simulink library "GenericINSLibrary"  (R2020b)
settings: Solver=VariableStepAuto  StartTime=0.0  StopTime=10.0  RelTol=1e-3
libraries: simulink x44
(part 3 of 6)

== system GenericINSLibrary/Empty Bus Sensor Fusion No Bias Estimation/GNSS6 ==
  Bus Creator : BusCreator  Inputs=1
  Bus Creator1 : BusCreator  Inputs=3
  Bus Creator2 : BusCreator  Inputs=3
  Bus Creator3 : BusCreator  Inputs=4
  Constant71 : Constant  Value=[0;0;0]  OutDataTypeStr=double
  Constant72 : Constant  OutDataTypeStr=double
  Constant73 : Constant  OutDataTypeStr=double
  Constant74 : Constant  OutDataTypeStr=double
  Constant{75..78} (4 alike) : Constant  Value=0  OutDataTypeStr=double
  Signal Specification : SignalSpecification  OutDataTypeStr=double  Unit=m  Dimensions=3
  Signal Specification{1..3,7} (4 alike) : SignalSpecification  OutDataTypeStr=double  Unit=m  Dimensions=1
  Signal Specification4 : SignalSpecification  OutDataTypeStr=double  Unit=s  Dimensions=1
  Signal Specification5 : SignalSpecification  OutDataTypeStr=double  Unit=rad  Dimensions=1
  Signal Specification6 : SignalSpecification  OutDataTypeStr=double  Unit=rad  Dimensions=1
  busGNSS : Outport
  wires:
  Bus Creator1/1 -> busGNSS/1
  Signal Specification4/1 -> Bus Creator3/1  "timestamp"
  Constant75/1 -> Signal Specification4/1
  Signal Specification/1 -> Bus Creator/1  "positionBodyToSensor"
  Signal Specification2/1 -> Bus Creator2/2  "east"
  Constant74/1 -> Signal Specification3/1
  Bus Creator/1 -> Bus Creator1/1  "alignment"
  Signal Specification3/1 -> Bus Creator2/3  "down"
  Bus Creator3/1 -> Bus Creator1/3  "measurement"
  Bus Creator2/1 -> Bus Creator1/2  "standardDeviation"
  Signal Specification5/1 -> Bus Creator3/2  "latitude"
  Constant78/1 -> Signal Specification7/1
  Signal Specification7/1 -> Bus Creator3/4  "altitude"
  Constant73/1 -> Signal Specification2/1
  Constant71/1 -> Signal Specification/1
  Constant76/1 -> Signal Specification5/1
  Constant77/1 -> Signal Specification6/1
  Signal Specification1/1 -> Bus Creator2/1  "north"
  Constant72/1 -> Signal Specification1/1
  Signal Specification6/1 -> Bus Creator3/3  "longitude"

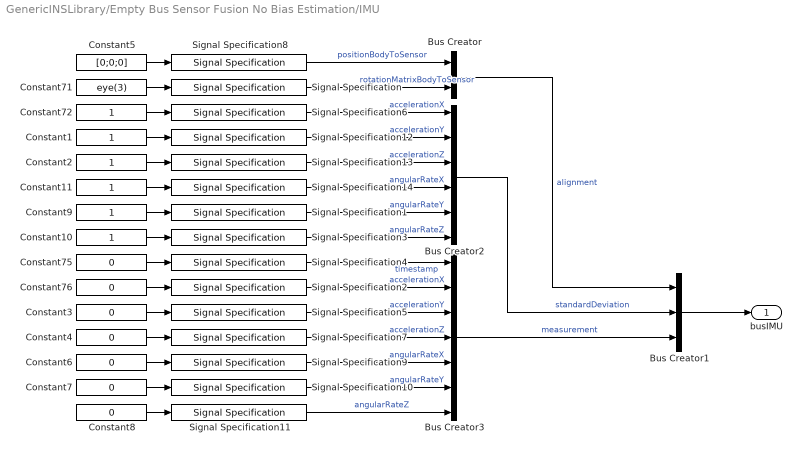
== system GenericINSLibrary/Empty Bus Sensor Fusion No Bias Estimation/IMU ==
  Bus Creator : BusCreator  Inputs=2
  Bus Creator1 : BusCreator  Inputs=3
  Bus Creator2 : BusCreator  Inputs=6
  Bus Creator3 : BusCreator  Inputs=7
  Constant{1..2,9..11,72} (6 alike) : Constant  OutDataTypeStr=double
  Constant{3..4,6..8,75..76} (7 alike) : Constant  Value=0  OutDataTypeStr=double
  Constant5 : Constant  Value=[0;0;0]  OutDataTypeStr=double
  Constant71 : Constant  Value=eye(3)  OutDataTypeStr=double
  Signal Specification : SignalSpecification  OutDataTypeStr=double  Dimensions=[3 3]
  Signal Specification{1,3,9..11,14} (6 alike) : SignalSpecification  OutDataTypeStr=double  Unit=rad/s  Dimensions=1
  Signal Specification{2,5..7,12..13} (6 alike) : SignalSpecification  OutDataTypeStr=double  Unit=m/s^2  Dimensions=1
  Signal Specification4 : SignalSpecification  OutDataTypeStr=double  Unit=s  Dimensions=1
  Signal Specification8 : SignalSpecification  OutDataTypeStr=double  Unit=m  Dimensions=3
  busIMU : Outport
  wires:
  Constant4/1 -> Signal Specification7/1
  Constant2/1 -> Signal Specification13/1
  Bus Creator1/1 -> busIMU/1
  Signal Specification4/1 -> Bus Creator3/1  "timestamp"
  Constant75/1 -> Signal Specification4/1
  Signal Specification/1 -> Bus Creator/2  "rotationMatrixBodyToSensor"
  Bus Creator/1 -> Bus Creator1/1  "alignment"
  Bus Creator3/1 -> Bus Creator1/3  "measurement"
  Bus Creator2/1 -> Bus Creator1/2  "standardDeviation"
  Constant71/1 -> Signal Specification/1
  Constant76/1 -> Signal Specification2/1
  Constant72/1 -> Signal Specification6/1
  Signal Specification2/1 -> Bus Creator3/2  "accelerationX"
  Constant1/1 -> Signal Specification12/1
  Constant3/1 -> Signal Specification5/1
  Signal Specification8/1 -> Bus Creator/1  "positionBodyToSensor"
  Constant5/1 -> Signal Specification8/1
  Signal Specification5/1 -> Bus Creator3/3  "accelerationY"
  Signal Specification7/1 -> Bus Creator3/4  "accelerationZ"
  Constant6/1 -> Signal Specification9/1
  Signal Specification9/1 -> Bus Creator3/5  "angularRateX"
  Constant7/1 -> Signal Specification10/1
  Constant8/1 -> Signal Specification11/1
  Signal Specification10/1 -> Bus Creator3/6  "angularRateY"
  Signal Specification11/1 -> Bus Creator3/7  "angularRateZ"
  Signal Specification3/1 -> Bus Creator2/6  "angularRateZ"
  Signal Specification1/1 -> Bus Creator2/5  "angularRateY"
  Signal Specification14/1 -> Bus Creator2/4  "angularRateX"
  Signal Specification13/1 -> Bus Creator2/3  "accelerationZ"
  Signal Specification12/1 -> Bus Creator2/2  "accelerationY"
  Signal Specification6/1 -> Bus Creator2/1  "accelerationX"
  Constant9/1 -> Signal Specification1/1
  Constant11/1 -> Signal Specification14/1
  Constant10/1 -> Signal Specification3/1

== system GenericINSLibrary/Empty Bus Sensor Fusion No Bias Estimation/InitialStandardDeviation ==
  Bus Creator2 : BusCreator  Inputs=9
  Constant{86..94} (9 alike) : Constant  OutDataTypeStr=double
  Signal Specification16 : SignalSpecification  OutDataTypeStr=double  Unit=m/s  Dimensions=1
  Signal Specification23 : SignalSpecification  OutDataTypeStr=double  Unit=m/s  Dimensions=1
  Signal Specification24 : SignalSpecification  OutDataTypeStr=double  Unit=m/s  Dimensions=1
  Signal Specification{25..27,29..30} (5 alike) : SignalSpecification  OutDataTypeStr=double  Unit=rad  Dimensions=1
  Signal Specification28 : SignalSpecification  OutDataTypeStr=double  Unit=m  Dimensions=1
  initialStandardDeviation : Outport
  wires:
  Signal Specification25/1 -> Bus Creator2/7  "orientationVectorX"
  Signal Specification23/1 -> Bus Creator2/5  "velocityV"
  Constant90/1 -> Signal Specification29/1
  Constant94/1 -> Signal Specification30/1
  Constant89/1 -> Signal Specification25/1
  Signal Specification16/1 -> Bus Creator2/4  "velocityU"
  Signal Specification26/1 -> Bus Creator2/1  "latitude"
  Constant88/1 -> Signal Specification24/1
  Signal Specification27/1 -> Bus Creator2/2  "longitude"
  Constant87/1 -> Signal Specification23/1
  Signal Specification24/1 -> Bus Creator2/6  "velocityW"
  Constant86/1 -> Signal Specification16/1
  Constant93/1 -> Signal Specification28/1
  Constant92/1 -> Signal Specification27/1
  Constant91/1 -> Signal Specification26/1
  Signal Specification28/1 -> Bus Creator2/3  "altitude"
  Bus Creator2/1 -> initialStandardDeviation/1  "standardDeviation"
  Signal Specification30/1 -> Bus Creator2/9  "orientationVectorZ"
  Signal Specification29/1 -> Bus Creator2/8  "orientationVectorY"

== system GenericINSLibrary/Empty Bus Sensor Fusion No Bias Estimation/InitialState ==
  Bus Creator1 : BusCreator  Inputs=9
  Constant{71..79} (9 alike) : Constant  Value=0  OutDataTypeStr=double
  Signal Specification1 : SignalSpecification  OutDataTypeStr=double  Unit=m/s  Dimensions=1
  Signal Specification2 : SignalSpecification  OutDataTypeStr=double  Unit=m/s  Dimensions=1
  Signal Specification3 : SignalSpecification  OutDataTypeStr=double  Unit=m/s  Dimensions=1
  Signal Specification{4..6,8..9} (5 alike) : SignalSpecification  OutDataTypeStr=double  Unit=rad  Dimensions=1
  Signal Specification7 : SignalSpecification  OutDataTypeStr=double  Unit=m  Dimensions=1
  initialState : Outport
  wires:
  Signal Specification4/1 -> Bus Creator1/7  "roll"
  Signal Specification6/1 -> Bus Creator1/2  "longitude"
  Constant73/1 -> Signal Specification3/1
  Constant79/1 -> Signal Specification9/1
  Signal Specification9/1 -> Bus Creator1/9  "yaw"
  Signal Specification2/1 -> Bus Creator1/5  "velocityV"
  Constant71/1 -> Signal Specification1/1
  Constant75/1 -> Signal Specification8/1
  Signal Specification5/1 -> Bus Creator1/1  "latitude"
  Signal Specification7/1 -> Bus Creator1/3  "altitude"
  Signal Specification8/1 -> Bus Creator1/8  "pitch"
  Signal Specification3/1 -> Bus Creator1/6  "velocityW"
  Signal Specification1/1 -> Bus Creator1/4  "velocityU"
  Constant72/1 -> Signal Specification2/1
  Constant77/1 -> Signal Specification6/1
  Constant76/1 -> Signal Specification5/1
  Bus Creator1/1 -> initialState/1
  Constant78/1 -> Signal Specification7/1
  Constant74/1 -> Signal Specification4/1

== system GenericINSLibrary/Empty Bus Sensor Fusion No Bias Estimation/SOG1 ==
  Bus Creator : BusCreator  Inputs=1
  Bus Creator1 : BusCreator  Inputs=3
  Bus Creator2 : BusCreator  Inputs=1
  Bus Creator3 : BusCreator  Inputs=2
  Constant71 : Constant  Value=[0;0;0]  OutDataTypeStr=double
  Constant72 : Constant  OutDataTypeStr=double
  Constant75 : Constant  Value=0  OutDataTypeStr=double
  Constant76 : Constant  Value=0  OutDataTypeStr=double
  Signal Specification : SignalSpecification  OutDataTypeStr=double  Unit=m  Dimensions=3
  Signal Specification1 : SignalSpecification  OutDataTypeStr=double  Unit=m/s  Dimensions=1
  Signal Specification2 : SignalSpecification  OutDataTypeStr=double  Unit=m/s  Dimensions=1
  Signal Specification4 : SignalSpecification  OutDataTypeStr=double  Unit=s  Dimensions=1
  busSOG : Outport
  wires:
  Bus Creator1/1 -> busSOG/1
  Signal Specification4/1 -> Bus Creator3/1  "timestamp"
  Constant75/1 -> Signal Specification4/1
  Signal Specification/1 -> Bus Creator/1  "positionBodyToSensor"
  Bus Creator/1 -> Bus Creator1/1  "alignment"
  Bus Creator3/1 -> Bus Creator1/3  "measurement"
  Bus Creator2/1 -> Bus Creator1/2  "standardDeviation"
  Constant71/1 -> Signal Specification/1
  Constant76/1 -> Signal Specification2/1
  Signal Specification1/1 -> Bus Creator2/1  "speedOverGround"
  Constant72/1 -> Signal Specification1/1
  Signal Specification2/1 -> Bus Creator3/2  "speedOverGround"

== system GenericINSLibrary/Empty Bus Sensor Fusion No Bias Estimation/SOG2 ==
  Bus Creator : BusCreator  Inputs=1
  Bus Creator1 : BusCreator  Inputs=3
  Bus Creator2 : BusCreator  Inputs=1
  Bus Creator3 : BusCreator  Inputs=2
  Constant71 : Constant  Value=[0;0;0]  OutDataTypeStr=double
  Constant72 : Constant  OutDataTypeStr=double
  Constant75 : Constant  Value=0  OutDataTypeStr=double
  Constant76 : Constant  Value=0  OutDataTypeStr=double
  Signal Specification : SignalSpecification  OutDataTypeStr=double  Unit=m  Dimensions=3
  Signal Specification1 : SignalSpecification  OutDataTypeStr=double  Unit=m/s  Dimensions=1
  Signal Specification2 : SignalSpecification  OutDataTypeStr=double  Unit=m/s  Dimensions=1
  Signal Specification4 : SignalSpecification  OutDataTypeStr=double  Unit=s  Dimensions=1
  busSOG : Outport
  wires:
  Signal Specification2/1 -> Bus Creator3/2  "speedOverGround"
  Constant72/1 -> Signal Specification1/1
  Signal Specification1/1 -> Bus Creator2/1  "speedOverGround"
  Constant76/1 -> Signal Specification2/1
  Constant71/1 -> Signal Specification/1
  Bus Creator2/1 -> Bus Creator1/2  "standardDeviation"
  Bus Creator3/1 -> Bus Creator1/3  "measurement"
  Bus Creator/1 -> Bus Creator1/1  "alignment"
  Signal Specification/1 -> Bus Creator/1  "positionBodyToSensor"
  Constant75/1 -> Signal Specification4/1
  Signal Specification4/1 -> Bus Creator3/1  "timestamp"
  Bus Creator1/1 -> busSOG/1

== system GenericINSLibrary/Empty Bus Sensor Fusion No Bias Estimation/SOG3 ==
  Bus Creator : BusCreator  Inputs=1
  Bus Creator1 : BusCreator  Inputs=3
  Bus Creator2 : BusCreator  Inputs=1
  Bus Creator3 : BusCreator  Inputs=2
  Constant71 : Constant  Value=[0;0;0]  OutDataTypeStr=double
  Constant72 : Constant  OutDataTypeStr=double
  Constant75 : Constant  Value=0  OutDataTypeStr=double
  Constant76 : Constant  Value=0  OutDataTypeStr=double
  Signal Specification : SignalSpecification  OutDataTypeStr=double  Unit=m  Dimensions=3
  Signal Specification1 : SignalSpecification  OutDataTypeStr=double  Unit=m/s  Dimensions=1
  Signal Specification2 : SignalSpecification  OutDataTypeStr=double  Unit=m/s  Dimensions=1
  Signal Specification4 : SignalSpecification  OutDataTypeStr=double  Unit=s  Dimensions=1
  busSOG : Outport
  wires:
  Bus Creator1/1 -> busSOG/1
  Signal Specification4/1 -> Bus Creator3/1  "timestamp"
  Constant75/1 -> Signal Specification4/1
  Signal Specification/1 -> Bus Creator/1  "positionBodyToSensor"
  Bus Creator/1 -> Bus Creator1/1  "alignment"
  Bus Creator3/1 -> Bus Creator1/3  "measurement"
  Bus Creator2/1 -> Bus Creator1/2  "standardDeviation"
  Constant71/1 -> Signal Specification/1
  Constant76/1 -> Signal Specification2/1
  Signal Specification1/1 -> Bus Creator2/1  "speedOverGround"
  Constant72/1 -> Signal Specification1/1
  Signal Specification2/1 -> Bus Creator3/2  "speedOverGround"

== system GenericINSLibrary/Empty Bus Sensor Fusion No Bias Estimation/SOG4 ==
  Bus Creator : BusCreator  Inputs=1
  Bus Creator1 : BusCreator  Inputs=3
  Bus Creator2 : BusCreator  Inputs=1
  Bus Creator3 : BusCreator  Inputs=2
  Constant71 : Constant  Value=[0;0;0]  OutDataTypeStr=double
  Constant72 : Constant  OutDataTypeStr=double
  Constant75 : Constant  Value=0  OutDataTypeStr=double
  Constant76 : Constant  Value=0  OutDataTypeStr=double
  Signal Specification : SignalSpecification  OutDataTypeStr=double  Unit=m  Dimensions=3
  Signal Specification1 : SignalSpecification  OutDataTypeStr=double  Unit=m/s  Dimensions=1
  Signal Specification2 : SignalSpecification  OutDataTypeStr=double  Unit=m/s  Dimensions=1
  Signal Specification4 : SignalSpecification  OutDataTypeStr=double  Unit=s  Dimensions=1
  busSOG : Outport
  wires:
  Signal Specification2/1 -> Bus Creator3/2  "speedOverGround"
  Constant72/1 -> Signal Specification1/1
  Signal Specification1/1 -> Bus Creator2/1  "speedOverGround"
  Constant76/1 -> Signal Specification2/1
  Constant71/1 -> Signal Specification/1
  Bus Creator2/1 -> Bus Creator1/2  "standardDeviation"
  Bus Creator3/1 -> Bus Creator1/3  "measurement"
  Bus Creator/1 -> Bus Creator1/1  "alignment"
  Signal Specification/1 -> Bus Creator/1  "positionBodyToSensor"
  Constant75/1 -> Signal Specification4/1
  Signal Specification4/1 -> Bus Creator3/1  "timestamp"
  Bus Creator1/1 -> busSOG/1

== system GenericINSLibrary/Empty Bus Sensor Fusion No Bias Estimation/SOG5 ==
  Bus Creator : BusCreator  Inputs=1
  Bus Creator1 : BusCreator  Inputs=3
  Bus Creator2 : BusCreator  Inputs=1
  Bus Creator3 : BusCreator  Inputs=2
  Constant71 : Constant  Value=[0;0;0]  OutDataTypeStr=double
  Constant72 : Constant  OutDataTypeStr=double
  Constant75 : Constant  Value=0  OutDataTypeStr=double
  Constant76 : Constant  Value=0  OutDataTypeStr=double
  Signal Specification : SignalSpecification  OutDataTypeStr=double  Unit=m  Dimensions=3
  Signal Specification1 : SignalSpecification  OutDataTypeStr=double  Unit=m/s  Dimensions=1
  Signal Specification2 : SignalSpecification  OutDataTypeStr=double  Unit=m/s  Dimensions=1
  Signal Specification4 : SignalSpecification  OutDataTypeStr=double  Unit=s  Dimensions=1
  busSOG : Outport
  wires:
  Bus Creator1/1 -> busSOG/1
  Signal Specification4/1 -> Bus Creator3/1  "timestamp"
  Constant75/1 -> Signal Specification4/1
  Signal Specification/1 -> Bus Creator/1  "positionBodyToSensor"
  Bus Creator/1 -> Bus Creator1/1  "alignment"
  Bus Creator3/1 -> Bus Creator1/3  "measurement"
  Bus Creator2/1 -> Bus Creator1/2  "standardDeviation"
  Constant71/1 -> Signal Specification/1
  Constant76/1 -> Signal Specification2/1
  Signal Specification1/1 -> Bus Creator2/1  "speedOverGround"
  Constant72/1 -> Signal Specification1/1
  Signal Specification2/1 -> Bus Creator3/2  "speedOverGround"

== system GenericINSLibrary/Empty Bus Sensor Fusion No Bias Estimation/SOG6 ==
  Bus Creator : BusCreator  Inputs=1
  Bus Creator1 : BusCreator  Inputs=3
  Bus Creator2 : BusCreator  Inputs=1
  Bus Creator3 : BusCreator  Inputs=2
  Constant71 : Constant  Value=[0;0;0]  OutDataTypeStr=double
  Constant72 : Constant  OutDataTypeStr=double
  Constant75 : Constant  Value=0  OutDataTypeStr=double
  Constant76 : Constant  Value=0  OutDataTypeStr=double
  Signal Specification : SignalSpecification  OutDataTypeStr=double  Unit=m  Dimensions=3
  Signal Specification1 : SignalSpecification  OutDataTypeStr=double  Unit=m/s  Dimensions=1
  Signal Specification2 : SignalSpecification  OutDataTypeStr=double  Unit=m/s  Dimensions=1
  Signal Specification4 : SignalSpecification  OutDataTypeStr=double  Unit=s  Dimensions=1
  busSOG : Outport
  wires:
  Signal Specification2/1 -> Bus Creator3/2  "speedOverGround"
  Constant72/1 -> Signal Specification1/1
  Signal Specification1/1 -> Bus Creator2/1  "speedOverGround"
  Constant76/1 -> Signal Specification2/1
  Constant71/1 -> Signal Specification/1
  Bus Creator2/1 -> Bus Creator1/2  "standardDeviation"
  Bus Creator3/1 -> Bus Creator1/3  "measurement"
  Bus Creator/1 -> Bus Creator1/1  "alignment"
  Signal Specification/1 -> Bus Creator/1  "positionBodyToSensor"
  Constant75/1 -> Signal Specification4/1
  Signal Specification4/1 -> Bus Creator3/1  "timestamp"
  Bus Creator1/1 -> busSOG/1

== system GenericINSLibrary/Empty Bus Sensor Fusion No Bias Estimation/VelocityXY1 ==
  Bus Creator : BusCreator  Inputs=2
  Bus Creator1 : BusCreator  Inputs=3
  Bus Creator2 : BusCreator  Inputs=2
  Bus Creator3 : BusCreator  Inputs=3
  Constant1 : Constant  OutDataTypeStr=double
  Constant3 : Constant  Value=0  OutDataTypeStr=double
  Constant5 : Constant  Value=[0;0;0]  OutDataTypeStr=double
  Constant71 : Constant  Value=eye(3)  OutDataTypeStr=double
  Constant72 : Constant  OutDataTypeStr=double
  Constant75 : Constant  Value=0  OutDataTypeStr=double
  Constant76 : Constant  Value=0  OutDataTypeStr=double
  Signal Specification : SignalSpecification  OutDataTypeStr=double  Dimensions=[3 3]
  Signal Specification{1..3,5} (4 alike) : SignalSpecification  OutDataTypeStr=double  Unit=m/s  Dimensions=1
  Signal Specification4 : SignalSpecification  OutDataTypeStr=double  Unit=s  Dimensions=1
  Signal Specification8 : SignalSpecification  OutDataTypeStr=double  Unit=m  Dimensions=3
  busVelocityXY : Outport
  wires:
  Bus Creator1/1 -> busVelocityXY/1
  Signal Specification4/1 -> Bus Creator3/1  "timestamp"
  Constant75/1 -> Signal Specification4/1
  Signal Specification/1 -> Bus Creator/2  "rotationMatrixBodyToSensor"
  Bus Creator/1 -> Bus Creator1/1  "alignment"
  Bus Creator3/1 -> Bus Creator1/3  "measurement"
  Bus Creator2/1 -> Bus Creator1/2  "standardDeviation"
  Constant71/1 -> Signal Specification/1
  Constant76/1 -> Signal Specification2/1
  Signal Specification1/1 -> Bus Creator2/1  "velocityX"
  Constant72/1 -> Signal Specification1/1
  Signal Specification2/1 -> Bus Creator3/2  "velocityX"
  Constant1/1 -> Signal Specification3/1
  Signal Specification3/1 -> Bus Creator2/2  "velocityY"
  Signal Specification5/1 -> Bus Creator3/3  "velocityY"
  Constant3/1 -> Signal Specification5/1
  Signal Specification8/1 -> Bus Creator/1  "positionBodyToSensor"
  Constant5/1 -> Signal Specification8/1

== system GenericINSLibrary/Empty Bus Sensor Fusion No Bias Estimation/VelocityXY2 ==
  Bus Creator : BusCreator  Inputs=2
  Bus Creator1 : BusCreator  Inputs=3
  Bus Creator2 : BusCreator  Inputs=2
  Bus Creator3 : BusCreator  Inputs=3
  Constant1 : Constant  OutDataTypeStr=double
  Constant3 : Constant  Value=0  OutDataTypeStr=double
  Constant5 : Constant  Value=[0;0;0]  OutDataTypeStr=double
  Constant71 : Constant  Value=eye(3)  OutDataTypeStr=double
  Constant72 : Constant  OutDataTypeStr=double
  Constant75 : Constant  Value=0  OutDataTypeStr=double
  Constant76 : Constant  Value=0  OutDataTypeStr=double
  Signal Specification : SignalSpecification  OutDataTypeStr=double  Dimensions=[3 3]
  Signal Specification{1..3,5} (4 alike) : SignalSpecification  OutDataTypeStr=double  Unit=m/s  Dimensions=1
  Signal Specification4 : SignalSpecification  OutDataTypeStr=double  Unit=s  Dimensions=1
  Signal Specification8 : SignalSpecification  OutDataTypeStr=double  Unit=m  Dimensions=3
  busVelocityXY : Outport
  wires:
  Constant5/1 -> Signal Specification8/1
  Signal Specification8/1 -> Bus Creator/1  "positionBodyToSensor"
  Constant3/1 -> Signal Specification5/1
  Signal Specification5/1 -> Bus Creator3/3  "velocityY"
  Signal Specification3/1 -> Bus Creator2/2  "velocityY"
  Constant1/1 -> Signal Specification3/1
  Signal Specification2/1 -> Bus Creator3/2  "velocityX"
  Constant72/1 -> Signal Specification1/1
  Signal Specification1/1 -> Bus Creator2/1  "velocityX"
  Constant76/1 -> Signal Specification2/1
  Constant71/1 -> Signal Specification/1
  Bus Creator2/1 -> Bus Creator1/2  "standardDeviation"
  Bus Creator3/1 -> Bus Creator1/3  "measurement"
  Bus Creator/1 -> Bus Creator1/1  "alignment"
  Signal Specification/1 -> Bus Creator/2  "rotationMatrixBodyToSensor"
  Constant75/1 -> Signal Specification4/1
  Signal Specification4/1 -> Bus Creator3/1  "timestamp"
  Bus Creator1/1 -> busVelocityXY/1

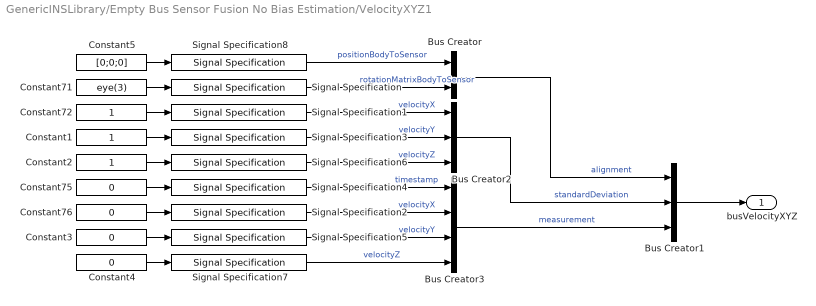
== system GenericINSLibrary/Empty Bus Sensor Fusion No Bias Estimation/VelocityXYZ1 ==
  Bus Creator : BusCreator  Inputs=2
  Bus Creator1 : BusCreator  Inputs=3
  Bus Creator2 : BusCreator  Inputs=3
  Bus Creator3 : BusCreator  Inputs=4
  Constant1 : Constant  OutDataTypeStr=double
  Constant2 : Constant  OutDataTypeStr=double
  Constant{3..4,75..76} (4 alike) : Constant  Value=0  OutDataTypeStr=double
  Constant5 : Constant  Value=[0;0;0]  OutDataTypeStr=double
  Constant71 : Constant  Value=eye(3)  OutDataTypeStr=double
  Constant72 : Constant  OutDataTypeStr=double
  Signal Specification : SignalSpecification  OutDataTypeStr=double  Dimensions=[3 3]
  Signal Specification{1..3,5..7} (6 alike) : SignalSpecification  OutDataTypeStr=double  Unit=m/s  Dimensions=1
  Signal Specification4 : SignalSpecification  OutDataTypeStr=double  Unit=s  Dimensions=1
  Signal Specification8 : SignalSpecification  OutDataTypeStr=double  Unit=m  Dimensions=3
  busVelocityXYZ : Outport
  wires:
  Constant5/1 -> Signal Specification8/1
  Signal Specification8/1 -> Bus Creator/1  "positionBodyToSensor"
  Constant3/1 -> Signal Specification5/1
  Signal Specification5/1 -> Bus Creator3/3  "velocityY"
  Signal Specification3/1 -> Bus Creator2/2  "velocityY"
  Constant1/1 -> Signal Specification3/1
  Signal Specification2/1 -> Bus Creator3/2  "velocityX"
  Constant72/1 -> Signal Specification1/1
  Signal Specification1/1 -> Bus Creator2/1  "velocityX"
  Constant76/1 -> Signal Specification2/1
  Constant71/1 -> Signal Specification/1
  Bus Creator2/1 -> Bus Creator1/2  "standardDeviation"
  Bus Creator3/1 -> Bus Creator1/3  "measurement"
  Bus Creator/1 -> Bus Creator1/1  "alignment"
  Signal Specification/1 -> Bus Creator/2  "rotationMatrixBodyToSensor"
  Constant75/1 -> Signal Specification4/1
  Signal Specification4/1 -> Bus Creator3/1  "timestamp"
  Bus Creator1/1 -> busVelocityXYZ/1
  Constant2/1 -> Signal Specification6/1
  Signal Specification6/1 -> Bus Creator2/3  "velocityZ"
  Constant4/1 -> Signal Specification7/1
  Signal Specification7/1 -> Bus Creator3/4  "velocityZ"

== system GenericINSLibrary/Empty Bus Sensor Fusion No Bias Estimation/VelocityXYZ2 ==
  Bus Creator : BusCreator  Inputs=2
  Bus Creator1 : BusCreator  Inputs=3
  Bus Creator2 : BusCreator  Inputs=3
  Bus Creator3 : BusCreator  Inputs=4
  Constant1 : Constant  OutDataTypeStr=double
  Constant2 : Constant  OutDataTypeStr=double
  Constant{3..4,75..76} (4 alike) : Constant  Value=0  OutDataTypeStr=double
  Constant5 : Constant  Value=[0;0;0]  OutDataTypeStr=double
  Constant71 : Constant  Value=eye(3)  OutDataTypeStr=double
  Constant72 : Constant  OutDataTypeStr=double
  Signal Specification : SignalSpecification  OutDataTypeStr=double  Dimensions=[3 3]
  Signal Specification{1..3,5..7} (6 alike) : SignalSpecification  OutDataTypeStr=double  Unit=m/s  Dimensions=1
  Signal Specification4 : SignalSpecification  OutDataTypeStr=double  Unit=s  Dimensions=1
  Signal Specification8 : SignalSpecification  OutDataTypeStr=double  Unit=m  Dimensions=3
  busVelocityXYZ : Outport
  wires:
  Signal Specification7/1 -> Bus Creator3/4  "velocityZ"
  Constant4/1 -> Signal Specification7/1
  Signal Specification6/1 -> Bus Creator2/3  "velocityZ"
  Constant2/1 -> Signal Specification6/1
  Bus Creator1/1 -> busVelocityXYZ/1
  Signal Specification4/1 -> Bus Creator3/1  "timestamp"
  Constant75/1 -> Signal Specification4/1
  Signal Specification/1 -> Bus Creator/2  "rotationMatrixBodyToSensor"
  Bus Creator/1 -> Bus Creator1/1  "alignment"
  Bus Creator3/1 -> Bus Creator1/3  "measurement"
  Bus Creator2/1 -> Bus Creator1/2  "standardDeviation"
  Constant71/1 -> Signal Specification/1
  Constant76/1 -> Signal Specification2/1
  Signal Specification1/1 -> Bus Creator2/1  "velocityX"
  Constant72/1 -> Signal Specification1/1
  Signal Specification2/1 -> Bus Creator3/2  "velocityX"
  Constant1/1 -> Signal Specification3/1
  Signal Specification3/1 -> Bus Creator2/2  "velocityY"
  Signal Specification5/1 -> Bus Creator3/3  "velocityY"
  Constant3/1 -> Signal Specification5/1
  Signal Specification8/1 -> Bus Creator/1  "positionBodyToSensor"
  Constant5/1 -> Signal Specification8/1

== system GenericINSLibrary/Sensor Fusion/AHRS1 ==
  AHRS : Inport
  Abs : Abs
  Bus Selector : BusSelector  OutputSignals=measurement.timestamp
  Bus Selector1 : BusSelector  OutputSignals=measurement.roll,measurement.pitch,measurement.yaw  OutputAsBus=on
  Bus Selector2 : BusSelector  OutputSignals=standardDeviation  OutputAsBus=on
  Bus Selector3 : BusSelector  OutputSignals=alignment
  Bus Selector5 : BusSelector  OutputSignals=rotationMatrixBodyToSensor
  Bus to Vector : BusToVector
  Data Type Conversion : DataTypeConversion  OutDataTypeStr=double
  Detect Increase : simulink/Logic and Bit Operations/Detect Increase  vinit=0.0  OutDataTypeStr=boolean
  Reshape1 : Reshape  OutputDimensionality=Customize  OutputDimensions=[3 1]
  Reshape3 : Reshape  OutputDimensionality=Customize  OutputDimensions=[3 1]
  Reshape4 : Reshape  OutputDimensionality=Customize  OutputDimensions=[3 3]
  Vector Concatenate : Concatenate
  data : Outport
  stdDev : Outport  Port=2
  sensorOrientation : Outport  Port=3
  wires:
  Reshape4/1 -> sensorOrientation/1
  Bus Selector5/1 -> Reshape4/1  "<rotationMatrixBodyToSensor>"
  Reshape1/1 -> stdDev/1
  Reshape3/1 -> Vector Concatenate/2
  Bus Selector3/1 -> Bus Selector5/1  "<alignment>"
  Abs/1 -> Reshape1/1
  Bus Selector2/1 -> Abs/1
  Vector Concatenate/1 -> data/1
  Bus to Vector/1 -> Reshape3/1
  Bus Selector1/1 -> Bus to Vector/1
  Detect Increase/1 -> Data Type Conversion/1
  Data Type Conversion/1 -> Vector Concatenate/1
  Bus Selector/1 -> Detect Increase/1  "<timestamp>"
  AHRS/1 -> Bus Selector/1, Bus Selector1/1, Bus Selector2/1, Bus Selector3/1

== system GenericINSLibrary/Sensor Fusion/AHRS2 ==
  AHRS : Inport
  Abs : Abs
  Bus Selector : BusSelector  OutputSignals=measurement.timestamp
  Bus Selector1 : BusSelector  OutputSignals=measurement.roll,measurement.pitch,measurement.yaw  OutputAsBus=on
  Bus Selector2 : BusSelector  OutputSignals=standardDeviation  OutputAsBus=on
  Bus Selector3 : BusSelector  OutputSignals=alignment
  Bus Selector5 : BusSelector  OutputSignals=rotationMatrixBodyToSensor
  Bus to Vector : BusToVector
  Data Type Conversion : DataTypeConversion  OutDataTypeStr=double
  Detect Increase : simulink/Logic and Bit Operations/Detect Increase  vinit=0.0  OutDataTypeStr=boolean
  Reshape1 : Reshape  OutputDimensionality=Customize  OutputDimensions=[3 1]
  Reshape3 : Reshape  OutputDimensionality=Customize  OutputDimensions=[3 1]
  Reshape4 : Reshape  OutputDimensionality=Customize  OutputDimensions=[3 3]
  Vector Concatenate : Concatenate
  data : Outport
  stdDev : Outport  Port=2
  sensorOrientation : Outport  Port=3
  wires:
  AHRS/1 -> Bus Selector3/1, Bus Selector2/1, Bus Selector1/1, Bus Selector/1
  Bus Selector/1 -> Detect Increase/1  "<timestamp>"
  Data Type Conversion/1 -> Vector Concatenate/1
  Detect Increase/1 -> Data Type Conversion/1
  Bus Selector1/1 -> Bus to Vector/1
  Bus to Vector/1 -> Reshape3/1
  Vector Concatenate/1 -> data/1
  Bus Selector2/1 -> Abs/1
  Abs/1 -> Reshape1/1
  Bus Selector3/1 -> Bus Selector5/1  "<alignment>"
  Reshape3/1 -> Vector Concatenate/2
  Reshape1/1 -> stdDev/1
  Bus Selector5/1 -> Reshape4/1  "<rotationMatrixBodyToSensor>"
  Reshape4/1 -> sensorOrientation/1

== system GenericINSLibrary/Sensor Fusion/Compass1 ==
  Compass : Inport
  Abs : Abs
  Bus Selector : BusSelector  OutputSignals=measurement.timestamp
  Bus Selector1 : BusSelector  OutputSignals=measurement.yaw
  Bus Selector2 : BusSelector  OutputSignals=standardDeviation  OutputAsBus=on
  Bus Selector3 : BusSelector  OutputSignals=alignment
  Bus Selector5 : BusSelector  OutputSignals=rotationMatrixBodyToSensor
  Data Type Conversion : DataTypeConversion  OutDataTypeStr=double
  Detect Increase : simulink/Logic and Bit Operations/Detect Increase  vinit=0.0  OutDataTypeStr=boolean
  Reshape4 : Reshape  OutputDimensionality=Customize  OutputDimensions=[3 3]
  Vector Concatenate : Concatenate
  data : Outport
  stdDev : Outport  Port=2
  sensorOrientation : Outport  Port=3
  wires:
  Compass/1 -> Bus Selector3/1, Bus Selector2/1, Bus Selector1/1, Bus Selector/1
  Bus Selector/1 -> Detect Increase/1  "<timestamp>"
  Data Type Conversion/1 -> Vector Concatenate/1
  Detect Increase/1 -> Data Type Conversion/1
  Bus Selector1/1 -> Vector Concatenate/2  "<yaw>"
  Vector Concatenate/1 -> data/1
  Bus Selector2/1 -> Abs/1
  Bus Selector3/1 -> Bus Selector5/1  "<alignment>"
  Abs/1 -> stdDev/1
  Bus Selector5/1 -> Reshape4/1  "<rotationMatrixBodyToSensor>"
  Reshape4/1 -> sensorOrientation/1

== system GenericINSLibrary/Sensor Fusion/Compass2 ==
  Compass : Inport
  Abs : Abs
  Bus Selector : BusSelector  OutputSignals=measurement.timestamp
  Bus Selector1 : BusSelector  OutputSignals=measurement.yaw
  Bus Selector2 : BusSelector  OutputSignals=standardDeviation  OutputAsBus=on
  Bus Selector3 : BusSelector  OutputSignals=alignment
  Bus Selector5 : BusSelector  OutputSignals=rotationMatrixBodyToSensor
  Data Type Conversion : DataTypeConversion  OutDataTypeStr=double
  Detect Increase : simulink/Logic and Bit Operations/Detect Increase  vinit=0.0  OutDataTypeStr=boolean
  Reshape4 : Reshape  OutputDimensionality=Customize  OutputDimensions=[3 3]
  Vector Concatenate : Concatenate
  data : Outport
  stdDev : Outport  Port=2
  sensorOrientation : Outport  Port=3
  wires:
  Reshape4/1 -> sensorOrientation/1
  Bus Selector5/1 -> Reshape4/1  "<rotationMatrixBodyToSensor>"
  Abs/1 -> stdDev/1
  Bus Selector3/1 -> Bus Selector5/1  "<alignment>"
  Bus Selector2/1 -> Abs/1
  Vector Concatenate/1 -> data/1
  Bus Selector1/1 -> Vector Concatenate/2  "<yaw>"
  Detect Increase/1 -> Data Type Conversion/1
  Data Type Conversion/1 -> Vector Concatenate/1
  Bus Selector/1 -> Detect Increase/1  "<timestamp>"
  Compass/1 -> Bus Selector/1, Bus Selector1/1, Bus Selector2/1, Bus Selector3/1

== system GenericINSLibrary/Sensor Fusion/GNSS1 ==
  GNSS : Inport
  Abs : Abs
  Bus Selector : BusSelector  OutputSignals=measurement.timestamp
  Bus Selector1 : BusSelector  OutputSignals=measurement.latitude,measurement.longitude,measurement.altitude  OutputAsBus=on
  Bus Selector2 : BusSelector  OutputSignals=standardDeviation  OutputAsBus=on
  Bus Selector3 : BusSelector  OutputSignals=alignment
  Bus Selector4 : BusSelector  OutputSignals=positionBodyToSensor
  Bus to Vector : BusToVector
  Data Type Conversion : DataTypeConversion  OutDataTypeStr=double
  Detect Increase : simulink/Logic and Bit Operations/Detect Increase  vinit=0.0  OutDataTypeStr=boolean
  Reshape1 : Reshape  OutputDimensionality=Customize  OutputDimensions=[3 1]
  Reshape2 : Reshape  OutputDimensionality=Customize  OutputDimensions=[3 1]
  Reshape3 : Reshape  OutputDimensionality=Customize  OutputDimensions=[3 1]
  Vector Concatenate : Concatenate
  data : Outport
  stdDev : Outport  Port=2
  sensorPosition : Outport  Port=3
  wires:
  Reshape2/1 -> sensorPosition/1
  Reshape1/1 -> stdDev/1
  Reshape3/1 -> Vector Concatenate/2
  Bus Selector4/1 -> Reshape2/1  "<positionBodyToSensor>"
  Bus Selector3/1 -> Bus Selector4/1  "<alignment>"
  Abs/1 -> Reshape1/1
  Bus Selector2/1 -> Abs/1
  Vector Concatenate/1 -> data/1
  Bus to Vector/1 -> Reshape3/1
  Bus Selector1/1 -> Bus to Vector/1
  Detect Increase/1 -> Data Type Conversion/1
  Data Type Conversion/1 -> Vector Concatenate/1
  Bus Selector/1 -> Detect Increase/1  "<timestamp>"
  GNSS/1 -> Bus Selector/1, Bus Selector1/1, Bus Selector2/1, Bus Selector3/1

== system GenericINSLibrary/Sensor Fusion/GNSS2 ==
  GNSS : Inport
  Abs : Abs
  Bus Selector : BusSelector  OutputSignals=measurement.timestamp
  Bus Selector1 : BusSelector  OutputSignals=measurement.latitude,measurement.longitude,measurement.altitude  OutputAsBus=on
  Bus Selector2 : BusSelector  OutputSignals=standardDeviation  OutputAsBus=on
  Bus Selector3 : BusSelector  OutputSignals=alignment
  Bus Selector4 : BusSelector  OutputSignals=positionBodyToSensor
  Bus to Vector : BusToVector
  Data Type Conversion : DataTypeConversion  OutDataTypeStr=double
  Detect Increase : simulink/Logic and Bit Operations/Detect Increase  vinit=0.0  OutDataTypeStr=boolean
  Reshape1 : Reshape  OutputDimensionality=Customize  OutputDimensions=[3 1]
  Reshape2 : Reshape  OutputDimensionality=Customize  OutputDimensions=[3 1]
  Reshape3 : Reshape  OutputDimensionality=Customize  OutputDimensions=[3 1]
  Vector Concatenate : Concatenate
  data : Outport
  stdDev : Outport  Port=2
  sensorPosition : Outport  Port=3
  wires:
  GNSS/1 -> Bus Selector3/1, Bus Selector2/1, Bus Selector1/1, Bus Selector/1
  Bus Selector/1 -> Detect Increase/1  "<timestamp>"
  Data Type Conversion/1 -> Vector Concatenate/1
  Detect Increase/1 -> Data Type Conversion/1
  Bus Selector1/1 -> Bus to Vector/1
  Bus to Vector/1 -> Reshape3/1
  Vector Concatenate/1 -> data/1
  Bus Selector2/1 -> Abs/1
  Abs/1 -> Reshape1/1
  Bus Selector3/1 -> Bus Selector4/1  "<alignment>"
  Bus Selector4/1 -> Reshape2/1  "<positionBodyToSensor>"
  Reshape3/1 -> Vector Concatenate/2
  Reshape1/1 -> stdDev/1
  Reshape2/1 -> sensorPosition/1

== system GenericINSLibrary/Sensor Fusion/GNSS3 ==
  GNSS : Inport
  Abs : Abs
  Bus Selector : BusSelector  OutputSignals=measurement.timestamp
  Bus Selector1 : BusSelector  OutputSignals=measurement.latitude,measurement.longitude,measurement.altitude  OutputAsBus=on
  Bus Selector2 : BusSelector  OutputSignals=standardDeviation  OutputAsBus=on
  Bus Selector3 : BusSelector  OutputSignals=alignment
  Bus Selector4 : BusSelector  OutputSignals=positionBodyToSensor
  Bus to Vector : BusToVector
  Data Type Conversion : DataTypeConversion  OutDataTypeStr=double
  Detect Increase : simulink/Logic and Bit Operations/Detect Increase  vinit=0.0  OutDataTypeStr=boolean
  Reshape1 : Reshape  OutputDimensionality=Customize  OutputDimensions=[3 1]
  Reshape2 : Reshape  OutputDimensionality=Customize  OutputDimensions=[3 1]
  Reshape3 : Reshape  OutputDimensionality=Customize  OutputDimensions=[3 1]
  Vector Concatenate : Concatenate
  data : Outport
  stdDev : Outport  Port=2
  sensorPosition : Outport  Port=3
  wires:
  GNSS/1 -> Bus Selector3/1, Bus Selector2/1, Bus Selector1/1, Bus Selector/1
  Bus Selector/1 -> Detect Increase/1  "<timestamp>"
  Data Type Conversion/1 -> Vector Concatenate/1
  Detect Increase/1 -> Data Type Conversion/1
  Bus Selector1/1 -> Bus to Vector/1
  Bus to Vector/1 -> Reshape3/1
  Vector Concatenate/1 -> data/1
  Bus Selector2/1 -> Abs/1
  Abs/1 -> Reshape1/1
  Bus Selector3/1 -> Bus Selector4/1  "<alignment>"
  Bus Selector4/1 -> Reshape2/1  "<positionBodyToSensor>"
  Reshape3/1 -> Vector Concatenate/2
  Reshape1/1 -> stdDev/1
  Reshape2/1 -> sensorPosition/1

== system GenericINSLibrary/Sensor Fusion/GNSS4 ==
  GNSS : Inport
  Abs : Abs
  Bus Selector : BusSelector  OutputSignals=measurement.timestamp
  Bus Selector1 : BusSelector  OutputSignals=measurement.latitude,measurement.longitude,measurement.altitude  OutputAsBus=on
  Bus Selector2 : BusSelector  OutputSignals=standardDeviation  OutputAsBus=on
  Bus Selector3 : BusSelector  OutputSignals=alignment
  Bus Selector4 : BusSelector  OutputSignals=positionBodyToSensor
  Bus to Vector : BusToVector
  Data Type Conversion : DataTypeConversion  OutDataTypeStr=double
  Detect Increase : simulink/Logic and Bit Operations/Detect Increase  vinit=0.0  OutDataTypeStr=boolean
  Reshape1 : Reshape  OutputDimensionality=Customize  OutputDimensions=[3 1]
  Reshape2 : Reshape  OutputDimensionality=Customize  OutputDimensions=[3 1]
  Reshape3 : Reshape  OutputDimensionality=Customize  OutputDimensions=[3 1]
  Vector Concatenate : Concatenate
  data : Outport
  stdDev : Outport  Port=2
  sensorPosition : Outport  Port=3
  wires:
  Reshape2/1 -> sensorPosition/1
  Reshape1/1 -> stdDev/1
  Reshape3/1 -> Vector Concatenate/2
  Bus Selector4/1 -> Reshape2/1  "<positionBodyToSensor>"
  Bus Selector3/1 -> Bus Selector4/1  "<alignment>"
  Abs/1 -> Reshape1/1
  Bus Selector2/1 -> Abs/1
  Vector Concatenate/1 -> data/1
  Bus to Vector/1 -> Reshape3/1
  Bus Selector1/1 -> Bus to Vector/1
  Detect Increase/1 -> Data Type Conversion/1
  Data Type Conversion/1 -> Vector Concatenate/1
  Bus Selector/1 -> Detect Increase/1  "<timestamp>"
  GNSS/1 -> Bus Selector/1, Bus Selector1/1, Bus Selector2/1, Bus Selector3/1

== system GenericINSLibrary/Sensor Fusion/GNSS5 ==
  GNSS : Inport
  Abs : Abs
  Bus Selector : BusSelector  OutputSignals=measurement.timestamp
  Bus Selector1 : BusSelector  OutputSignals=measurement.latitude,measurement.longitude,measurement.altitude  OutputAsBus=on
  Bus Selector2 : BusSelector  OutputSignals=standardDeviation  OutputAsBus=on
  Bus Selector3 : BusSelector  OutputSignals=alignment
  Bus Selector4 : BusSelector  OutputSignals=positionBodyToSensor
  Bus to Vector : BusToVector
  Data Type Conversion : DataTypeConversion  OutDataTypeStr=double
  Detect Increase : simulink/Logic and Bit Operations/Detect Increase  vinit=0.0  OutDataTypeStr=boolean
  Reshape1 : Reshape  OutputDimensionality=Customize  OutputDimensions=[3 1]
  Reshape2 : Reshape  OutputDimensionality=Customize  OutputDimensions=[3 1]
  Reshape3 : Reshape  OutputDimensionality=Customize  OutputDimensions=[3 1]
  Vector Concatenate : Concatenate
  data : Outport
  stdDev : Outport  Port=2
  sensorPosition : Outport  Port=3
  wires:
  Reshape2/1 -> sensorPosition/1
  Reshape1/1 -> stdDev/1
  Reshape3/1 -> Vector Concatenate/2
  Bus Selector4/1 -> Reshape2/1  "<positionBodyToSensor>"
  Bus Selector3/1 -> Bus Selector4/1  "<alignment>"
  Abs/1 -> Reshape1/1
  Bus Selector2/1 -> Abs/1
  Vector Concatenate/1 -> data/1
  Bus to Vector/1 -> Reshape3/1
  Bus Selector1/1 -> Bus to Vector/1
  Detect Increase/1 -> Data Type Conversion/1
  Data Type Conversion/1 -> Vector Concatenate/1
  Bus Selector/1 -> Detect Increase/1  "<timestamp>"
  GNSS/1 -> Bus Selector/1, Bus Selector1/1, Bus Selector2/1, Bus Selector3/1

== system GenericINSLibrary/Sensor Fusion/GNSS6 ==
  GNSS : Inport
  Abs : Abs
  Bus Selector : BusSelector  OutputSignals=measurement.timestamp
  Bus Selector1 : BusSelector  OutputSignals=measurement.latitude,measurement.longitude,measurement.altitude  OutputAsBus=on
  Bus Selector2 : BusSelector  OutputSignals=standardDeviation  OutputAsBus=on
  Bus Selector3 : BusSelector  OutputSignals=alignment
  Bus Selector4 : BusSelector  OutputSignals=positionBodyToSensor
  Bus to Vector : BusToVector
  Data Type Conversion : DataTypeConversion  OutDataTypeStr=double
  Detect Increase : simulink/Logic and Bit Operations/Detect Increase  vinit=0.0  OutDataTypeStr=boolean
  Reshape1 : Reshape  OutputDimensionality=Customize  OutputDimensions=[3 1]
  Reshape2 : Reshape  OutputDimensionality=Customize  OutputDimensions=[3 1]
  Reshape3 : Reshape  OutputDimensionality=Customize  OutputDimensions=[3 1]
  Vector Concatenate : Concatenate
  data : Outport
  stdDev : Outport  Port=2
  sensorPosition : Outport  Port=3
  wires:
  GNSS/1 -> Bus Selector3/1, Bus Selector2/1, Bus Selector1/1, Bus Selector/1
  Bus Selector/1 -> Detect Increase/1  "<timestamp>"
  Data Type Conversion/1 -> Vector Concatenate/1
  Detect Increase/1 -> Data Type Conversion/1
  Bus Selector1/1 -> Bus to Vector/1
  Bus to Vector/1 -> Reshape3/1
  Vector Concatenate/1 -> data/1
  Bus Selector2/1 -> Abs/1
  Abs/1 -> Reshape1/1
  Bus Selector3/1 -> Bus Selector4/1  "<alignment>"
  Bus Selector4/1 -> Reshape2/1  "<positionBodyToSensor>"
  Reshape3/1 -> Vector Concatenate/2
  Reshape1/1 -> stdDev/1
  Reshape2/1 -> sensorPosition/1

== system GenericINSLibrary/Sensor Fusion/IMU ==
  IMU : Inport
  Abs : Abs
  Abs1 : Abs
  Bus Selector1 : BusSelector  OutputSignals=standardDeviation  OutputAsBus=on
  Bus Selector2 : BusSelector  OutputSignals=alignment
  Bus Selector3 : BusSelector  OutputSignals=positionBodyToSensor,rotationMatrixBodyToSensor
  Bus Selector6 : BusSelector  OutputSignals=measurement.timestamp
  Bus Selector7 : BusSelector  OutputSignals=measurement.accelerationX,measurement.accelerationY,measurement.accelerationZ,measurement.angularRateX,measurement.angularRateY,measurement.angularRateZ  OutputAsBus=on
  Bus to Vector2 : BusToVector
  Data Type Conversion : DataTypeConversion  OutDataTypeStr=double
  Detect Increase : simulink/Logic and Bit Operations/Detect Increase  vinit=0.0  OutDataTypeStr=boolean
  Enabled Subsystem : Subsystem  TreatAsAtomicUnit=on
  Reshape : Reshape  OutputDimensionality=Customize  OutputDimensions=[3 1]
  Reshape1 : Reshape  OutputDimensionality=Customize  OutputDimensions=[3 3]
  Reshape2 : Reshape  OutputDimensionality=Customize  OutputDimensions=[12 1]
  Reshape3 : Reshape  OutputDimensionality=Customize  OutputDimensions=[6 1]
  Vector Concatenate : Concatenate
  sampletime : Outport
  data : Outport  Port=2
  stdDev : Outport  Port=3
  sensorPosition : Outport  Port=4
  sensorOrientation : Outport  Port=5
  wires:
  Abs1/1 -> sampletime/1
  Reshape3/1 -> Vector Concatenate/2
  Reshape2/1 -> stdDev/1
  Reshape1/1 -> sensorOrientation/1
  Reshape/1 -> sensorPosition/1
  Bus Selector3/2 -> Reshape1/1  "<rotationMatrixBodyToSensor>"
  Bus Selector3/1 -> Reshape/1  "<positionBodyToSensor>"
  Bus Selector2/1 -> Bus Selector3/1  "<alignment>"
  Abs/1 -> Reshape2/1
  Bus Selector1/1 -> Abs/1
  Data Type Conversion/1 -> Vector Concatenate/1
  Detect Increase/1 -> Enabled Subsystem/Enable, Data Type Conversion/1
  Bus to Vector2/1 -> Reshape3/1
  Vector Concatenate/1 -> data/1
  IMU/1 -> Bus Selector7/1, Bus Selector6/1, Bus Selector1/1, Bus Selector2/1
  Enabled Subsystem/1(sampletime) -> Abs1/1
  Bus Selector6/1 -> Detect Increase/1, Enabled Subsystem/1(timestamp)  "<timestamp>"
  Bus Selector7/1 -> Bus to Vector2/1

== system GenericINSLibrary/Sensor Fusion/SOG1 ==
  SOG : Inport
  Abs1 : Abs
  Abs2 : Abs
  Bus Selector : BusSelector  OutputSignals=measurement.timestamp
  Bus Selector1 : BusSelector  OutputSignals=measurement
  Bus Selector2 : BusSelector  OutputSignals=standardDeviation
  Bus Selector3 : BusSelector  OutputSignals=alignment
  Bus Selector4 : BusSelector  OutputSignals=positionBodyToSensor
  Bus Selector5 : BusSelector  OutputSignals=speedOverGround
  Bus Selector6 : BusSelector  OutputSignals=speedOverGround
  Data Type Conversion : DataTypeConversion  OutDataTypeStr=double
  Detect Increase : simulink/Logic and Bit Operations/Detect Increase  vinit=0.0  OutDataTypeStr=boolean
  Reshape2 : Reshape  OutputDimensionality=Customize  OutputDimensions=[3 1]
  Vector Concatenate : Concatenate
  data : Outport
  stdDev : Outport  Port=2
  sensorPosition : Outport  Port=3
  wires:
  Bus Selector6/1 -> Abs2/1  "<speedOverGround>"
  Bus Selector2/1 -> Bus Selector6/1  "<standardDeviation>"
  Bus Selector5/1 -> Abs1/1  "<speedOverGround>"
  Abs1/1 -> Vector Concatenate/2
  Reshape2/1 -> sensorPosition/1
  Abs2/1 -> stdDev/1
  Bus Selector4/1 -> Reshape2/1  "<positionBodyToSensor>"
  Bus Selector3/1 -> Bus Selector4/1  "<alignment>"
  Vector Concatenate/1 -> data/1
  Bus Selector1/1 -> Bus Selector5/1  "<measurement>"
  Detect Increase/1 -> Data Type Conversion/1
  Data Type Conversion/1 -> Vector Concatenate/1
  Bus Selector/1 -> Detect Increase/1  "<timestamp>"
  SOG/1 -> Bus Selector/1, Bus Selector1/1, Bus Selector2/1, Bus Selector3/1

== system GenericINSLibrary/Sensor Fusion/SOG2 ==
  SOG : Inport
  Abs1 : Abs
  Abs2 : Abs
  Bus Selector : BusSelector  OutputSignals=measurement.timestamp
  Bus Selector1 : BusSelector  OutputSignals=measurement
  Bus Selector2 : BusSelector  OutputSignals=standardDeviation
  Bus Selector3 : BusSelector  OutputSignals=alignment
  Bus Selector4 : BusSelector  OutputSignals=positionBodyToSensor
  Bus Selector5 : BusSelector  OutputSignals=speedOverGround
  Bus Selector6 : BusSelector  OutputSignals=speedOverGround
  Data Type Conversion : DataTypeConversion  OutDataTypeStr=double
  Detect Increase : simulink/Logic and Bit Operations/Detect Increase  vinit=0.0  OutDataTypeStr=boolean
  Reshape2 : Reshape  OutputDimensionality=Customize  OutputDimensions=[3 1]
  Vector Concatenate : Concatenate
  data : Outport
  stdDev : Outport  Port=2
  sensorPosition : Outport  Port=3
  wires:
  SOG/1 -> Bus Selector3/1, Bus Selector2/1, Bus Selector1/1, Bus Selector/1
  Bus Selector/1 -> Detect Increase/1  "<timestamp>"
  Data Type Conversion/1 -> Vector Concatenate/1
  Detect Increase/1 -> Data Type Conversion/1
  Bus Selector1/1 -> Bus Selector5/1  "<measurement>"
  Vector Concatenate/1 -> data/1
  Bus Selector3/1 -> Bus Selector4/1  "<alignment>"
  Bus Selector4/1 -> Reshape2/1  "<positionBodyToSensor>"
  Abs2/1 -> stdDev/1
  Reshape2/1 -> sensorPosition/1
  Abs1/1 -> Vector Concatenate/2
  Bus Selector5/1 -> Abs1/1  "<speedOverGround>"
  Bus Selector2/1 -> Bus Selector6/1  "<standardDeviation>"
  Bus Selector6/1 -> Abs2/1  "<speedOverGround>"

== system GenericINSLibrary/Sensor Fusion/SOG3 ==
  SOG : Inport
  Abs1 : Abs
  Abs2 : Abs
  Bus Selector : BusSelector  OutputSignals=measurement.timestamp
  Bus Selector1 : BusSelector  OutputSignals=measurement
  Bus Selector2 : BusSelector  OutputSignals=standardDeviation
  Bus Selector3 : BusSelector  OutputSignals=alignment
  Bus Selector4 : BusSelector  OutputSignals=positionBodyToSensor
  Bus Selector5 : BusSelector  OutputSignals=speedOverGround
  Bus Selector6 : BusSelector  OutputSignals=speedOverGround
  Data Type Conversion : DataTypeConversion  OutDataTypeStr=double
  Detect Increase : simulink/Logic and Bit Operations/Detect Increase  vinit=0.0  OutDataTypeStr=boolean
  Reshape2 : Reshape  OutputDimensionality=Customize  OutputDimensions=[3 1]
  Vector Concatenate : Concatenate
  data : Outport
  stdDev : Outport  Port=2
  sensorPosition : Outport  Port=3
  wires:
  SOG/1 -> Bus Selector3/1, Bus Selector2/1, Bus Selector1/1, Bus Selector/1
  Bus Selector/1 -> Detect Increase/1  "<timestamp>"
  Data Type Conversion/1 -> Vector Concatenate/1
  Detect Increase/1 -> Data Type Conversion/1
  Bus Selector1/1 -> Bus Selector5/1  "<measurement>"
  Vector Concatenate/1 -> data/1
  Bus Selector3/1 -> Bus Selector4/1  "<alignment>"
  Bus Selector4/1 -> Reshape2/1  "<positionBodyToSensor>"
  Abs2/1 -> stdDev/1
  Reshape2/1 -> sensorPosition/1
  Abs1/1 -> Vector Concatenate/2
  Bus Selector5/1 -> Abs1/1  "<speedOverGround>"
  Bus Selector2/1 -> Bus Selector6/1  "<standardDeviation>"
  Bus Selector6/1 -> Abs2/1  "<speedOverGround>"

== system GenericINSLibrary/Sensor Fusion/SOG4 ==
  SOG : Inport
  Abs1 : Abs
  Abs2 : Abs
  Bus Selector : BusSelector  OutputSignals=measurement.timestamp
  Bus Selector1 : BusSelector  OutputSignals=measurement
  Bus Selector2 : BusSelector  OutputSignals=standardDeviation
  Bus Selector3 : BusSelector  OutputSignals=alignment
  Bus Selector4 : BusSelector  OutputSignals=positionBodyToSensor
  Bus Selector5 : BusSelector  OutputSignals=speedOverGround
  Bus Selector6 : BusSelector  OutputSignals=speedOverGround
  Data Type Conversion : DataTypeConversion  OutDataTypeStr=double
  Detect Increase : simulink/Logic and Bit Operations/Detect Increase  vinit=0.0  OutDataTypeStr=boolean
  Reshape2 : Reshape  OutputDimensionality=Customize  OutputDimensions=[3 1]
  Vector Concatenate : Concatenate
  data : Outport
  stdDev : Outport  Port=2
  sensorPosition : Outport  Port=3
  wires:
  Bus Selector6/1 -> Abs2/1  "<speedOverGround>"
  Bus Selector2/1 -> Bus Selector6/1  "<standardDeviation>"
  Bus Selector5/1 -> Abs1/1  "<speedOverGround>"
  Abs1/1 -> Vector Concatenate/2
  Reshape2/1 -> sensorPosition/1
  Abs2/1 -> stdDev/1
  Bus Selector4/1 -> Reshape2/1  "<positionBodyToSensor>"
  Bus Selector3/1 -> Bus Selector4/1  "<alignment>"
  Vector Concatenate/1 -> data/1
  Bus Selector1/1 -> Bus Selector5/1  "<measurement>"
  Detect Increase/1 -> Data Type Conversion/1
  Data Type Conversion/1 -> Vector Concatenate/1
  Bus Selector/1 -> Detect Increase/1  "<timestamp>"
  SOG/1 -> Bus Selector/1, Bus Selector1/1, Bus Selector2/1, Bus Selector3/1
